simulink model "AM_SITL"  (R2025b)
settings: Solver=VariableStepAuto  StartTime=0.0  StopTime=10.0  RelTol=1e-3
settings Model: Creator=eeman  LastModifiedBy=BillL

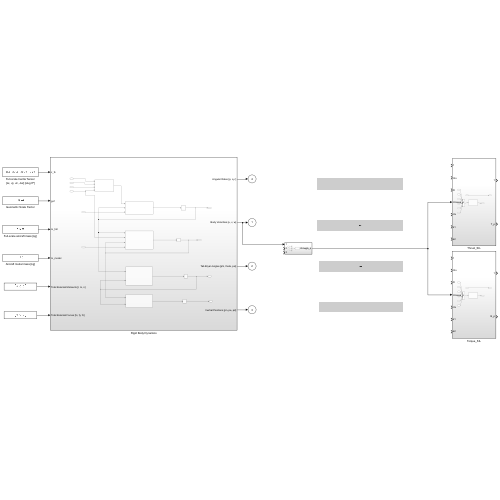
[thumbnail: Simulink's stored preview of the top-level diagram]
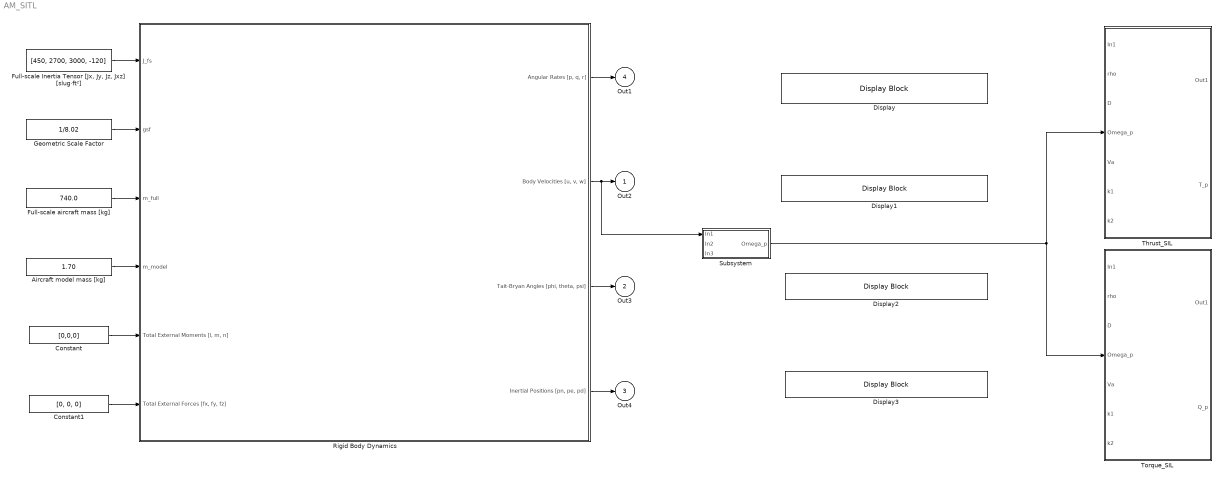
== system AM_SITL ==
  Aircraft model mass [kg] : Constant  Value=1.70
  Constant : Constant  Value=[0,0,0]
  Constant1 : Constant  Value=[0, 0, 0]
  Display{,1..3} (4 alike) : DisplayBlock  LabelPosition=Hide  Transparency=1  GridColor=[0.502, 0.502, 0.502]
  "Full-scale Inertia Tensor [Jx, Jy, Jz, Jxz] [slug·ft²]" : Constant  Value=[450, 2700, 3000, -120]
  Full-scale aircraft mass [kg] : Constant  Value=740.0
  Geometric Scale Factor : Constant  Value=1/8.02
  Rigid Body Dynamics : Subsystem
  Subsystem : Subsystem
  Thrust_SIL : Subsystem
  Torque_SIL : Subsystem
  Out2 : Outport
  Out3 : Outport  Port=2
  Out4 : Outport  Port=3
  Out1 : Outport  Port=4
  wires:
  "Full-scale Inertia Tensor [Jx, Jy, Jz, Jxz] [slug·ft²]"/1 -> Rigid Body Dynamics/1(J_fs)
  Geometric Scale Factor/1 -> Rigid Body Dynamics/2(gsf)
  Full-scale aircraft mass [kg]/1 -> Rigid Body Dynamics/3(m_full)
  Aircraft model mass [kg]/1 -> Rigid Body Dynamics/4(m_model)
  Constant/1 -> Rigid Body Dynamics/5("Total External Moments [l, m, n]")
  Constant1/1 -> Rigid Body Dynamics/6("Total External Forces [fx, fy, fz]")
  Rigid Body Dynamics/1("Angular Rates [p, q, r]") -> Out1/1
  Rigid Body Dynamics/3("Tait-Bryan Angles [phi, theta, psi]") -> Out3/1
  Rigid Body Dynamics/4("Inertial Positions [pn, pe, pd]") -> Out4/1
  Rigid Body Dynamics/2("Body Velocities [u, v, w]") -> Subsystem/1(In1), Out2/1
  Subsystem/1(Omega_p) -> Thrust_SIL/4(Omega_p), Torque_SIL/4(Omega_p)

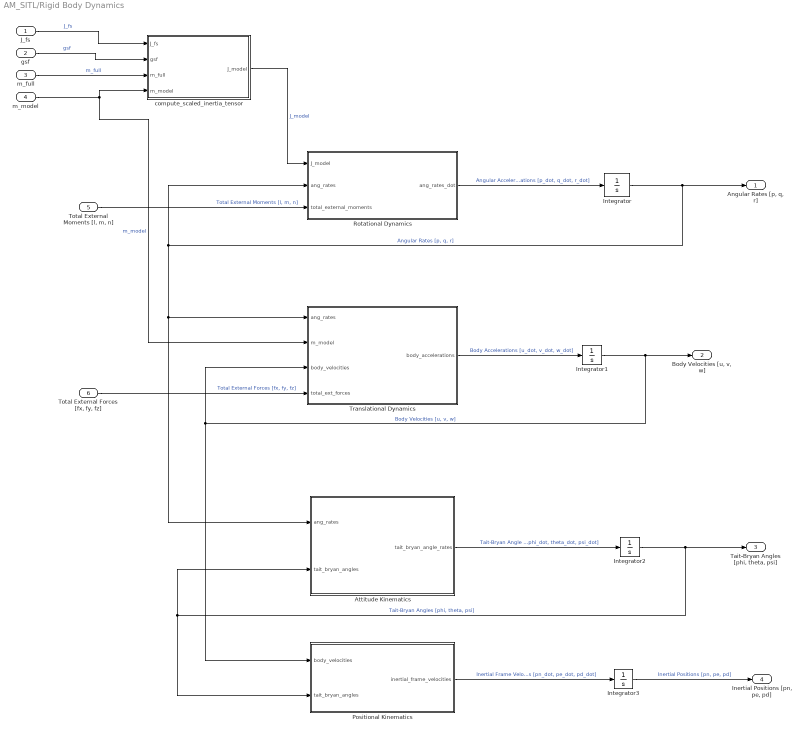
== system AM_SITL/Rigid Body Dynamics ==
  J_fs : Inport
  gsf : Inport  Port=2
  m_full : Inport  Port=3
  m_model : Inport  Port=4
  "Total External Moments [l, m, n]" : Inport  Port=5
  "Total External Forces [fx, fy, fz]" : Inport  Port=6
  Attitude Kinematics : MATLAB Function  TreatAsAtomicUnit=on
  Integrator{,1..3} (4 alike) : Integrator
  Positional Kinematics : MATLAB Function  TreatAsAtomicUnit=on
  Rotational Dynamics : MATLAB Function  TreatAsAtomicUnit=on
  Translational Dynamics : MATLAB Function  TreatAsAtomicUnit=on
  compute_scaled_inertia_tensor : MATLAB Function  TreatAsAtomicUnit=on
  "Angular Rates [p, q, r]" : Outport
  "Body Velocities [u, v, w]" : Outport  Port=2
  "Tait-Bryan Angles [phi, theta, psi]" : Outport  Port=3
  "Inertial Positions [pn, pe, pd]" : Outport  Port=4
  wires:
  gsf/1 -> compute_scaled_inertia_tensor/2(gsf)  "gsf"
  J_fs/1 -> compute_scaled_inertia_tensor/1(J_fs)  "J_fs"
  Translational Dynamics/1(body_accelerations) -> Integrator1/1  "Body Accelerations [u_dot, v_dot, w_dot]"
  Positional Kinematics/1(inertial_frame_velocities) -> Integrator3/1  "Inertial Frame Velocities [pn_dot, pe_dot, pd_dot]"
  Rotational Dynamics/1(ang_rates_dot) -> Integrator/1  "Angular Accelerations [p_dot, q_dot, r_dot]"
  m_full/1 -> compute_scaled_inertia_tensor/3(m_full)  "m_full"
  m_model/1 -> Translational Dynamics/2(m_model), compute_scaled_inertia_tensor/4(m_model)  "m_model"
  Attitude Kinematics/1(tait_bryan_angle_rates) -> Integrator2/1  "Tait-Bryan Angle Rates [phi_dot, theta_dot, psi_dot]"
  "Total External Moments [l, m, n]"/1 -> Rotational Dynamics/3(total_external_moments)  "Total External Moments [l, m, n]"
  Integrator3/1 -> "Inertial Positions [pn, pe, pd]"/1  "Inertial Positions [pn, pe, pd]"
  Integrator/1 -> "Angular Rates [p, q, r]"/1, Rotational Dynamics/2(ang_rates), Translational Dynamics/1(ang_rates), Attitude Kinematics/1(ang_rates)  "Angular Rates [p, q, r]"
  compute_scaled_inertia_tensor/1(J_model) -> Rotational Dynamics/1(J_model)  "J_model"
  Integrator2/1 -> "Tait-Bryan Angles [phi, theta, psi]"/1, Positional Kinematics/2(tait_bryan_angles), Attitude Kinematics/2(tait_bryan_angles)  "Tait-Bryan Angles [phi, theta, psi]"
  "Total External Forces [fx, fy, fz]"/1 -> Translational Dynamics/4(total_ext_forces)  "Total External Forces [fx, fy, fz]"
  Integrator1/1 -> "Body Velocities [u, v, w]"/1, Translational Dynamics/3(body_velocities), Positional Kinematics/1(body_velocities)  "Body Velocities [u, v, w]"

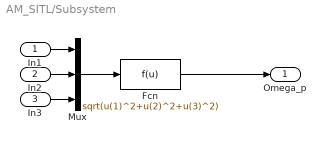
== system AM_SITL/Subsystem ==
  In1 : Inport
  In2 : Inport  Port=2
  In3 : Inport  Port=3
  Fcn : Fcn  Expr=sqrt(u(1)^2+u(2)^2+u(3)^2)
  Mux : Mux  Inputs=3
  Omega_p : Outport
  wires:
  In2/1 -> Mux/2
  In1/1 -> Mux/1
  In3/1 -> Mux/3
  Mux/1 -> Fcn/1
  Fcn/1 -> Omega_p/1

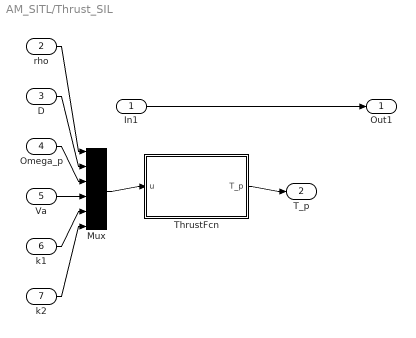
== system AM_SITL/Thrust_SIL ==
  In1 : Inport
  rho : Inport  Port=2
  D : Inport  Port=3
  Omega_p : Inport  Port=4
  Va : Inport  Port=5
  k1 : Inport  Port=6
  k2 : Inport  Port=7
  Mux : Mux  Inputs=6
  ThrustFcn : MATLAB Function  TreatAsAtomicUnit=on
  Out1 : Outport
  T_p : Outport  Port=2
  wires:
  In1/1 -> Out1/1
  rho/1 -> Mux/1
  D/1 -> Mux/2
  Omega_p/1 -> Mux/3
  Va/1 -> Mux/4
  k1/1 -> Mux/5
  k2/1 -> Mux/6
  Mux/1 -> ThrustFcn/1(u)
  ThrustFcn/1(T_p) -> T_p/1

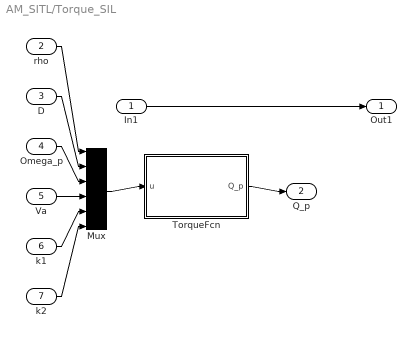
== system AM_SITL/Torque_SIL ==
  In1 : Inport
  rho : Inport  Port=2
  D : Inport  Port=3
  Omega_p : Inport  Port=4
  Va : Inport  Port=5
  k1 : Inport  Port=6
  k2 : Inport  Port=7
  Mux : Mux  Inputs=6
  TorqueFcn : MATLAB Function  TreatAsAtomicUnit=on
  Out1 : Outport
  Q_p : Outport  Port=2
  wires:
  In1/1 -> Out1/1
  rho/1 -> Mux/1
  D/1 -> Mux/2
  Omega_p/1 -> Mux/3
  Va/1 -> Mux/4
  k1/1 -> Mux/5
  k2/1 -> Mux/6
  Mux/1 -> TorqueFcn/1(u)
  TorqueFcn/1(Q_p) -> Q_p/1

== matlab function AM_SITL/Rigid Body Dynamics/Rotational Dynamics ==
  data: J_model input size=[1 4]; ang_rates input size=[1 3]; ang_rates_dot output size=[1 3]; total_external_moments input size=[1 3]
function ang_rates_dot = rotationalRGB(J_model, ang_rates, total_external_moments)
    
    % Clarifying vars used
    Jx = J_model(1);
    Jy = J_model(2);
    Jz = J_model(3);
    Jxz = J_model(4);
    p = ang_rates(1);
    q = ang_rates(2);
    r = ang_rates(3);
    l = total_external_moments(1);
    m = total_external_moments(2);
    n = total_external_moments(3);
    
    % Calculate gamma constants from Equation 9
    Gamma = Jx * Jz - Jxz^2;
    Gamma1 = (Jxz * (Jx - Jy + Jz)) / Gamma;
    Gamma2 = ((Jz * (Jz - Jy)) + Jxz^2) / Gamma;
    Gamma3 = Jz / Gamma;
    Gamma4 = Jxz / Gamma;
    Gamma5 = (Jz - Jx) / Jy;
    Gamma6 = Jxz / Jy;
    Gamma7 = ((Jx * (Jx - Jy)) + Jxz^2) / Gamma;
    Gamma8 = Jx / Gamma;
    
    % Equation 9
    p_dot = Gamma1*p*q - Gamma2*q*r + Gamma3*l + Gamma4*n;
    q_dot = Gamma5*p*r - Gamma6*(p^2 - r^2) + (1/Jy)*m;
    r_dot = Gamma7*p*q - Gamma1*q*r + Gamma4*l + Gamma8*n;
    
    ang_rates_dot = [p_dot, q_dot, r_dot];

end

== matlab function AM_SITL/Rigid Body Dynamics/compute_scaled_inertia_tensor ==
  data: J_fs input size=[1 4]; gsf input; J_model output size=[1 4]; m_full input; m_model input
function J_model = fcn(J_fs, gsf, m_full, m_model)
% This function calculates the scaled-down inertias for a model aircraft.
% It converts full-scale imperial inertias to SI units and applies a scaling factor.
%
% INPUTS:
%   J_fs array:
%       - Jx_full:   Full-scale roll inertia [slug·ft²]
%       - Jy_full:   Full-scale pitch inertia [slug·ft²]
%       - Jz_full:   Full-scale yaw inertia [slug·ft²]
%       - Jxz_full:  Full-scale product of inertia [slug·ft²]
%   mass array:
%       - m_full:    Full-scale aircraft mass [kg]
%       - m_model:   Model aircraft mass [kg]
%   gsf: Geometric scale factor (e.g., 1/8.02)
%
% OUTPUTS:
%   Jx: Scaled model roll inertia [kg·m²]
%   Jy: Scaled model pitch inertia [kg·m²]
%   Jz: Scaled model yaw inertia [kg·m²]
%   Jxz: Scaled model product of inertia [kg·m²]

% Unit conversion constant
slugft2_to_kgm2 = 1.35581795;

% Effective inertia scaling factor = (mass_ratio) * (length_ratio)^2
s = (m_model / m_full) * (gsf ^ 2);

% Convert full-scale inertias from imperial (slug·ft²) to SI (kg·m²)
Jx_full_SI = J_fs(1) * slugft2_to_kgm2;
Jy_full_SI = J_fs(2) * slugft2_to_kgm2;
Jz_full_SI = J_fs(3) * slugft2_to_kgm2;
Jxz_full_SI = J_fs(4) * slugft2_to_kgm2;

% Apply scaling to get the final model inertias in SI units
Jx = Jx_full_SI * s;
Jy = Jy_full_SI * s;
Jz = Jz_full_SI * s;
Jxz = Jxz_full_SI * s;

J_model = [Jx, Jy, Jz, Jxz];

end

== matlab function AM_SITL/Rigid Body Dynamics/Translational Dynamics ==
  data: ang_rates input size=[1 3]; m_model input; body_accelerations output size=[1 3]; body_velocities input size=[1 3]; total_ext_forces input size=[1 3]
function body_accelerations = translationalRGB(ang_rates, m_model, body_velocities, total_ext_forces)
    % Set up vars for clarity
    p = ang_rates(1);
    q = ang_rates(2);
    r = ang_rates(3);
    u = body_velocities(1);
    v = body_velocities(2);
    w = body_velocities(3);
    fx = total_ext_forces(1);
    fy = total_ext_forces(2);
    fz = total_ext_forces(3);
    mass = m_model;

    % Equation 6
    u_dot = r*v - q*w + fx/mass;
    v_dot = p*w - r*u + fy/mass;
    w_dot = q*u - p*v + fz/mass;

    % Return body accelerations
    body_accelerations = [u_dot, v_dot, w_dot];
end

== matlab function AM_SITL/Rigid Body Dynamics/Attitude Kinematics ==
  data: ang_rates input size=[1 3]; tait_bryan_angle_rates output size=[1 3]; tait_bryan_angles input size=[1 3]
function tait_bryan_angle_rates = attitude_kin(ang_rates, tait_bryan_angles)
    % Set up vars for clarity
    p = ang_rates(1);
    q = ang_rates(2);
    r = ang_rates(3);
    phi = tait_bryan_angles(1);
    theta = tait_bryan_angles(2);
    
    % Equation 4
    phi_dot   = p + q*sin(phi)*tan(theta) + r*cos(phi)*tan(theta);
    theta_dot = q*cos(phi) - r*sin(phi);
    psi_dot   = q*(sin(phi)/cos(theta)) + r*(cos(phi)/cos(theta));
    
    tait_bryan_angle_rates = [phi_dot, theta_dot, psi_dot];

end

== matlab function AM_SITL/Rigid Body Dynamics/Positional Kinematics ==
  data: body_velocities input size=[1 3]; inertial_frame_velocities output size=[1 3]; tait_bryan_angles input size=[1 3]
function inertial_frame_velocities = positional_kin(body_velocities, tait_bryan_angles)

    % Set up vars for clarity
    u = body_velocities(1);
    v = body_velocities(2);
    w = body_velocities(3);
    phi = tait_bryan_angles(1);
    theta = tait_bryan_angles(2);
    psi = tait_bryan_angles(3);

    % Rotation Matrix from Equation 1 (transposed for body-to-vehicle)
    R_b_v = [cos(theta)*cos(psi), sin(phi)*sin(theta)*cos(psi) - cos(phi)*sin(psi), cos(phi)*sin(theta)*cos(psi) + sin(phi)*sin(psi);
             cos(theta)*sin(psi), sin(phi)*sin(theta)*sin(psi) + cos(phi)*cos(psi), cos(phi)*sin(theta)*sin(psi) - sin(phi)*cos(psi);
             -1*sin(theta),         sin(phi)*cos(theta),                              cos(phi)*cos(theta)];

    % Equation 3 (outputs pn_dot, pe_dot, pd_dot)
    inertial_frame_velocities_col_vector = R_b_v * [u; v; w];
    inertial_frame_velocities = [inertial_frame_velocities_col_vector(1), inertial_frame_velocities_col_vector(2), inertial_frame_velocities_col_vector(3)];
end

== matlab function AM_SITL/Thrust_SIL/ThrustFcn ==
  data: u input; T_p output
function T_p = thrust_block(u)
rho = u(1); D = u(2); Omega_p = u(3); Va = u(4); k1 = u(5); k2 = u(6);
if Omega_p <= 0 || D <= 0
    J = 0; C_T = 0;
else
    J = (2*pi*Va) / (Omega_p*D);
    C_T = k1*J + k2*J^2;
end
T_p = (rho*D^4/(4*pi^2)) * Omega_p^2 * C_T;
end

== matlab function AM_SITL/Torque_SIL/TorqueFcn ==
  data: u input; Q_p output
function Q_p = torque_block(u)
rho = u(1); D = u(2); Omega_p = u(3); Va = u(4); k1 = u(5); k2 = u(6);
if Omega_p <= 0 || D <= 0
    J = 0; C_Q = 0;
else
    J = (2*pi*Va) / (Omega_p*D);
    C_Q = k1*J + k2*J^2;
end
Q_p = (rho*D^5/(4*pi^2)) * Omega_p^2 * C_Q;
end
